simulink model "VL53L1A1_Full"  (R2024b)
settings: Solver=FixedStepDiscrete  StartTime=0.0  StopTime=inf  RelTol=1e-3  EnableMultiTasking=on
PreLoadFcn:
  | addpath(genpath(pwd))
InitFcn:
  | addpath(genpath(pwd));
  | auto_program("VL53L1A1_Full");
  | STLINK_COMPORT = auto_COMPORT()
  | 
  | dialogPrms = get_param(gcs+"/VL53L1A1", 'DialogParameters');
  | dialogPrmNames = fieldnames(dialogPrms);
  | odr4 = get_param(gcs+"/VL53L1A1", dialogPrmNames{2});
  | odr4 = eval(odr4);
  | 
  | STM32_ODR = odr4
  | clearvars -except STLINK_COMPORT STLINK_DRIVE STM32_ODR
libraries: etargetslib x4, instrumentseriallib x3
settings Model: SimulationMode=accelerator  PacingRate=0.100000  ExtModeTrigDuration=10  Creator=JesseJabezArendse  LastModifiedBy=JesseJabezArendse
settings OptimizationCC: ReuseModelBlockBuffer=off  PassReuseOutputArgsAs=Individual arguments  ZeroExternalMemoryAtStartup=off  ZeroInternalMemoryAtStartup=off  MaxStackSize=64  OptimizationLevel=level1  OptimizationCustomize=off  EfficientTunableParamExpr=on
settings DebuggingCC: ParameterPrecisionLossMsg=none  ParameterTunabilityLossMsg=error
settings HardwareCC: ProdBitPerPointer=32  ProdBitPerSizeT=32  ProdBitPerPtrDiffT=32  ProdLargestAtomicInteger=Long  ProdLargestAtomicFloat=Double  ProdWordSize=32  ProdLongLongMode=on  ProdHWDeviceType=ARM Compatible->ARM Cortex
settings ModelReferenceCC: EnableParallelModelReferenceBuilds=on
settings SFSimCC: SimCustomHeaderCode="#include \"Core\\Inc\\main.h\""  SimParseCustomCode=off  MATLABDynamicMemAlloc=off  SimHardwareAcceleration=native
settings SFSimCC: SimUserSources=|
  | Core\Src\main.c
  | Core\Src\IKS02A1_Simulink.c
settings SFSimCC: SimUserIncludeDirs=|
  | Core\Inc\
  | Core\Src\
settings RTWCC: Description=Embedded Coder  SystemTargetFile=ert.tlc  TemplateMakefile=ert_default_tmf  RTWUseSimCustomCode=on  CustomHeaderCode="#include \"Core\\Inc\\main.h\""  Toolchain=GNU Tools for ARM Embedded Processors  BuildConfiguration=Specify  GPUComputeCapability=3.5
settings RTWCC: CustomInclude=|
  | Core\Inc\
  | Core\Src\
settings RTWCC: CustomSource=|
  | Core\Src\main.c
  | Core\Src\IKS02A1_Simulink.c
settings CodeAppCC: ForceParamTrailComments=on  IgnoreCustomStorageClasses=off  OperatorAnnotations=on  SimulinkDataObjDesc=on  SFDataObjDesc=on  InsertBlockDesc=on
settings ERTTargetCC: CodeReplacementLibrary=ARM Cortex-M  SupportContinuousTime=on  ExtModeTransport=3  ExtModeStaticAlloc=on  ExtModeStaticAllocSize=2000  ExtModeMexFile=ext_xcp  ExtModeIntrfLevel=Level2 - Open  InlinedParameterPlacement=Hierarchical  ERTCustomFileTemplate=example_file_process.tlc  DynamicArrayContainerType=coder::array

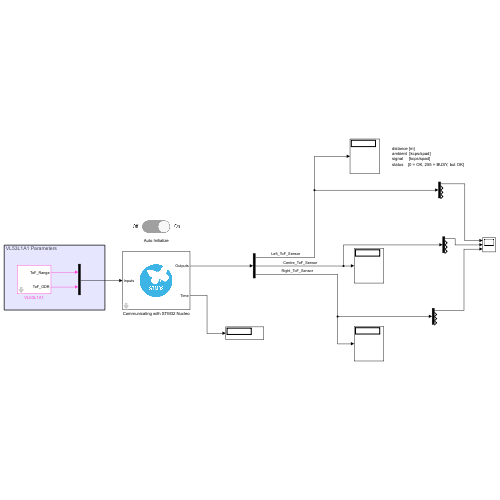
[thumbnail: Simulink's stored preview of the top-level diagram]
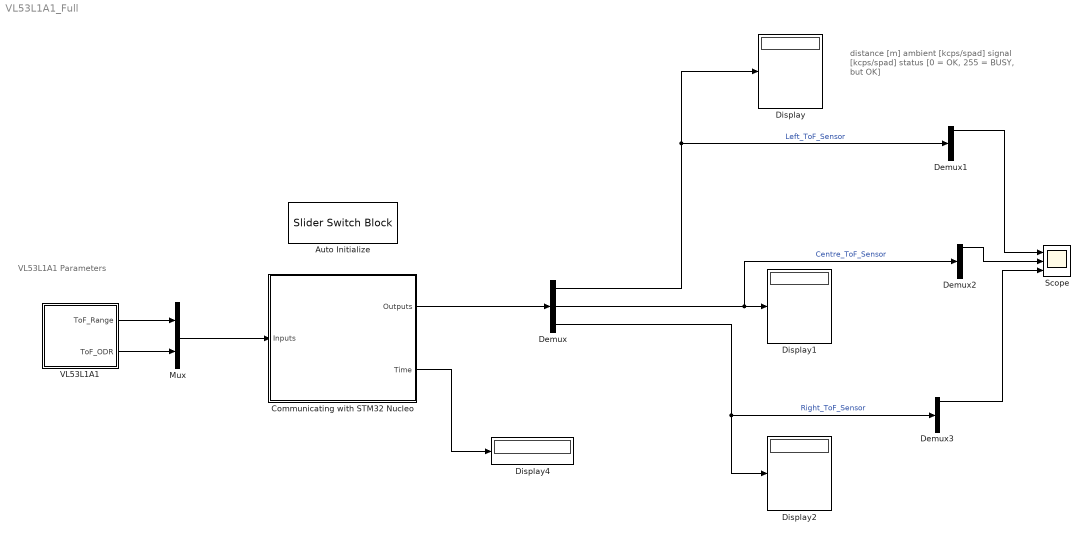
== system VL53L1A1_Full ==
  note: VL53L1A1 Parameters
  note: distance [m]
      | ambient [kcps/spad]
      | signal [kcps/spad]
      | status [0 = OK, 255 = BUSY, but OK]
  Auto Initialize : SliderSwitchBlock  LabelPosition=Hide
      settings: Values={{'Off', 'On'}, [0 1]}
  Communicating with STM32 Nucleo : Subsystem  mask{Auto_Initalize=1}
      mask prompts: Auto_Initalize "Automate Initialization?"
      mask TypeOptions Auto_Initalize: 1 | 0
      mask DialogControl Control1 Prompt: Block for communication between host machine and STM32 Nucleo F411RE
      mask Display: image('stm32_icon.png', [0,0,0,0,80,80]);
  Demux : Demux  Outputs=[4 4 4 ]
  Demux1 : Demux
  Demux2 : Demux
  Demux3 : Demux
  Display{,1..2,4} (4 alike) : Display
  Mux : Mux  Inputs=2
  Scope : Scope  NumInputPorts=3
  VL53L1A1 : Subsystem  mask{FSR_TOFOption=Long, ODR_TOFOption=10}
      mask prompts: FSR_TOFOption "Ranging Profile"; ODR_TOFOption "Output Data Rate (Hz)"
      mask init:
      | FSR_TOFVals = [1 , 2 , 3];
      |     FSR_TOF = FSR_TOFVals(FSR_TOFOption);
      |     
      |     ODR_TOFVals = [1 , 5, 10, 20, 30];
      |     ODR_TOF = ODR_TOFVals(ODR_TOFOption);
      mask TypeOptions FSR_TOFOption: Short | Medium | Long
      mask TypeOptions ODR_TOFOption: 1 | 5 | 10 | 20 | 30
      mask DialogControl DescGroupVar Prompt: Time of Flight Sensor 1x3
  wires:
  Demux/1 -> Demux1/1, Display/1  "Left_ToF_Sensor"
  Demux/2 -> Display1/1, Demux2/1  "Centre_ToF_Sensor"
  Demux/3 -> Display2/1, Demux3/1  "Right_ToF_Sensor"
  Demux1/1 -> Scope/1
  Demux2/1 -> Scope/2
  Demux3/1 -> Scope/3
  Communicating with STM32 Nucleo/1(Outputs) -> Demux/1
  Communicating with STM32 Nucleo/2(Time) -> Display4/1
  VL53L1A1/1(ToF_Range) -> Mux/1
  VL53L1A1/2(ToF_ODR) -> Mux/2
  Mux/1 -> Communicating with STM32 Nucleo/1(Inputs)

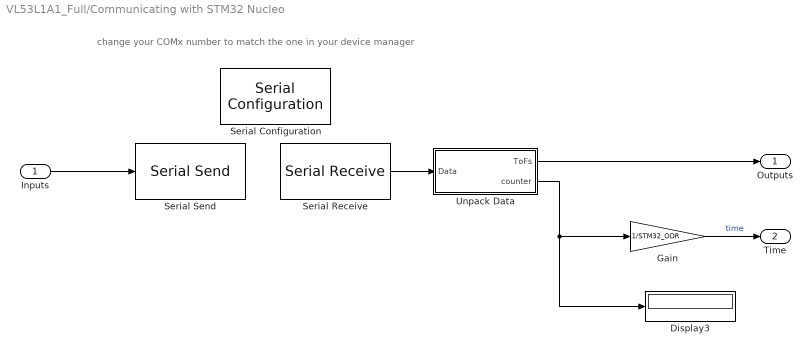
== system VL53L1A1_Full/Communicating with STM32 Nucleo ==
  note: change your COMx number to match the one in your device manager
  Inputs : Inport
  Display3 : Display
  Gain : Gain  Gain=1/STM32_ODR
  Serial Configuration : instrumentseriallib/Serial Configuration  Priority=-200000  PortSel=STLINK_COMPORT  Port=STLINK_COMPORT  ComPort=STLINK_COMPORT  BaudRate=1843200  DataBits=8  Parity=even  StopBits=2  ByteOrder=little-endian  FlowControl=none  Timeout=5  SimulateUsing=Interpreted execution  BlockInModel=on  aMode=1
      settings: LibrarySourceBlock=embeddedtargetslib/Host Communication/Serial Configuration
  Serial Receive : instrumentseriallib/Serial Receive  Priority=1  PortSel=STLINK_COMPORT  Port=STLINK_COMPORT  ComPort=STLINK_COMPORT  DataType=single  SaveDataType=uint8  ToggleHeader=on  Header='J_A'  ToggleDataSize=on  DataSize=[1 4*3+1]  ToggleTerminator=on  Terminator=Custom terminator  CustomTerminator='A_J'  InputFormat=Column major  EnableBlockingMode=on  ActionDataUnavailable=Output last received value  ActionWhenDataUnavailable=Output last received value  CustomValue=0  SampleTime=1/STM32_ODR  SimulateUsing=Interpreted execution  BlockInModel=on  aMode=1
      settings: LibrarySourceBlock=embeddedtargetslib/Host Communication/Serial Receive
  Serial Send : instrumentseriallib/Serial Send  Priority=1  PortSel=STLINK_COMPORT  Port=STLINK_COMPORT  ComPort=STLINK_COMPORT  Header='J_A'  Terminator=Custom terminator  CustomTerminator='A_J'  EnableBlockingMode=off  SimulateUsing=Interpreted execution  BlockInModel=on  aMode=1
      settings: LibrarySourceBlock=embeddedtargetslib/Host Communication/Serial Send
  Unpack Data : Subsystem
  Outputs : Outport
  Time : Outport  Port=2
  wires:
  Unpack Data/2(counter) -> Display3/1, Gain/1
  Gain/1 -> Time/1  "time"
  Unpack Data/1(ToFs) -> Outputs/1
  Serial Receive/1 -> Unpack Data/1(Data)
  Inputs/1 -> Serial Send/1

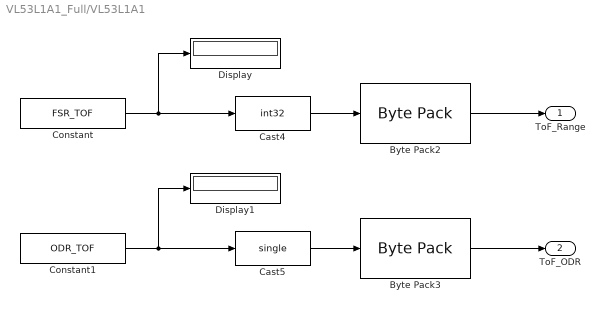
== system VL53L1A1_Full/VL53L1A1 ==
  Byte Pack2 : etargetslib/Byte Pack  datatypes={'int32'}  byteAlign=1
  Byte Pack3 : etargetslib/Byte Pack  datatypes={'single'}  byteAlign=1
  Cast4 : DataTypeConversion  OutDataTypeStr=int32  SaturateOnIntegerOverflow=off  RndMeth=Floor
  Cast5 : DataTypeConversion  OutDataTypeStr=single  SaturateOnIntegerOverflow=off  RndMeth=Floor
  Constant : Constant  Value=FSR_TOF
  Constant1 : Constant  Value=ODR_TOF
  Display : Display
  Display1 : Display
  ToF_Range : Outport
  ToF_ODR : Outport  Port=2
  wires:
  Constant/1 -> Cast4/1, Display/1
  Constant1/1 -> Cast5/1, Display1/1
  Cast4/1 -> Byte Pack2/1
  Cast5/1 -> Byte Pack3/1
  Byte Pack2/1 -> ToF_Range/1
  Byte Pack3/1 -> ToF_ODR/1

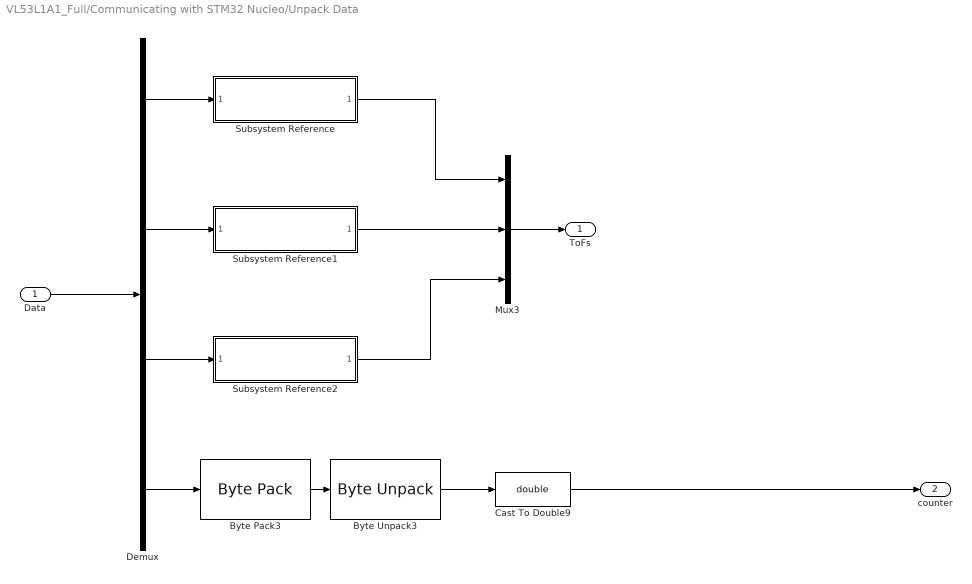
== system VL53L1A1_Full/Communicating with STM32 Nucleo/Unpack Data ==
  Data : Inport
  Byte Pack3 : etargetslib/Byte Pack  datatypes={'single'}  byteAlign=1
  Byte Unpack3 : etargetslib/Byte Unpack  dimensions={[1]}  datatypes={'uint32'}  byteAlign=1
      settings: LibrarySourceBlock=embeddedtargetslib/Host Communication/Byte Unpack
  Cast To Double9 : DataTypeConversion  OutDataTypeStr=double  SaturateOnIntegerOverflow=off  RndMeth=Floor
  Demux : Demux  Outputs=[4 4 4 1]
  Mux3 : Mux  Inputs=[4 4 4]
  Subsystem Reference : Subsystem  ReferencedSubsystem=unpack_ToF
  Subsystem Reference1 : Subsystem  ReferencedSubsystem=unpack_ToF
  Subsystem Reference2 : Subsystem  ReferencedSubsystem=unpack_ToF
  ToFs : Outport
  counter : Outport  Port=2
  wires:
  Mux3/1 -> ToFs/1
  Data/1 -> Demux/1
  Cast To Double9/1 -> counter/1
  Byte Unpack3/1 -> Cast To Double9/1
  Byte Pack3/1 -> Byte Unpack3/1
  Demux/4 -> Byte Pack3/1
  Demux/1 -> Subsystem Reference/1
  Demux/2 -> Subsystem Reference1/1
  Demux/3 -> Subsystem Reference2/1
  Subsystem Reference/1 -> Mux3/1
  Subsystem Reference1/1 -> Mux3/2
  Subsystem Reference2/1 -> Mux3/3
